simulink model "autoquet_simulink_expo_model"  (R2023b)
settings: Solver=FixedStepAuto  StartTime=0.0  StopTime=600  FixedStep=1e-4  RelTol=1e-3  EnableMultiTasking=on
libraries: svdutilitieslib x20, arduinolib x12, dspfdesign x2, arduinosensorlib x1
settings Model: ExtModeTrigDuration=2  Creator=doria  LastModifiedBy=doria
settings OptimizationCC: BlockReduction=off  EnhancedBackFolding=on  PassReuseOutputArgsAs=Individual arguments  ZeroExternalMemoryAtStartup=off  ZeroInternalMemoryAtStartup=off  MaxStackSize=64  OptimizeBlockOrder=speed  DifferentSizesBufferReuse=on  OptimizationCustomize=off  EfficientTunableParamExpr=on
settings DebuggingCC: MultiTaskCondExecSysMsg=warning  MultiTaskRateTransMsg=warning  ParameterTunabilityLossMsg=error
settings HardwareCC: ProdBitPerInt=16  ProdBitPerPointer=16  ProdBitPerSizeT=16  ProdBitPerPtrDiffT=16  ProdLargestAtomicFloat=None  ProdWordSize=8  ProdHWDeviceType=Atmel->AVR
settings ModelReferenceCC: UpdateModelReferenceTargets=Force
settings SFSimCC: MATLABDynamicMemAlloc=off
settings RTWCC: Description=Embedded Coder  SystemTargetFile=ert.tlc  HardwareBoard=Arduino Micro  TemplateMakefile=ert_default_tmf  Toolchain=Arduino AVR  BuildConfiguration=Faster Runs
settings CodeAppCC: ForceParamTrailComments=on  IgnoreCustomStorageClasses=off  OperatorAnnotations=on  SimulinkDataObjDesc=on  SFDataObjDesc=on  InsertBlockDesc=on
settings ERTTargetCC: SupportContinuousTime=on  SupportVariableSizeSignals=on  ExtModeTransport=3  ExtModeStaticAlloc=on  ExtModeAutomaticAllocSize=off  ExtModeStaticAllocSize=250  ExtModeMexFile=ext_xcp  ExtModeIntrfLevel=Level2 - Open

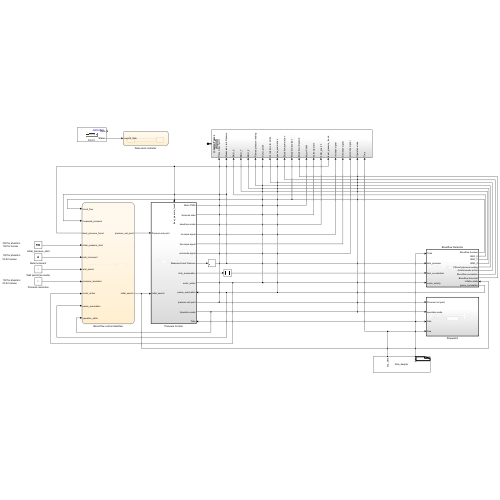
[thumbnail: Simulink's stored preview of the top-level diagram]
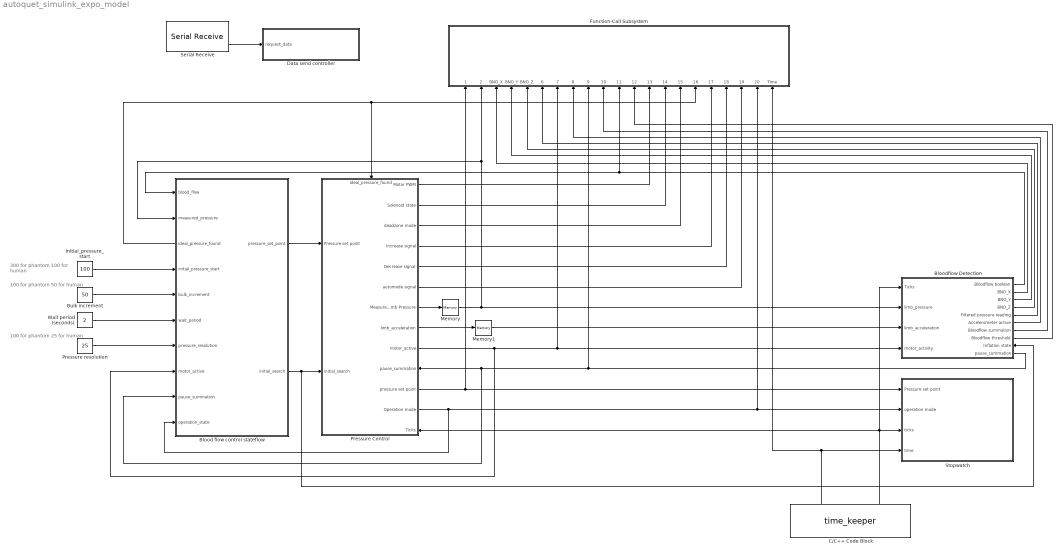
== system autoquet_simulink_expo_model ==
  note: 100 for phantom
      | 25 for human
  note: 100 for phantom
      | 50 for human
  note: 300 for phantom
      | 100 for human
  Blood flow control stateflow : Stateflow chart  TreatAsAtomicUnit=on
      settings: PortSchema="{\"entries\":[{\"content\":{\"sides\":[{\"content\":{\"connectorIds\":[\"In1\",\"In2\",\"Out3\",\"In4\",\"In5\",\"In6\",\"In7\",\"In3\",\"In9\",\"In8\"]},\"type\":\"ConnectorPlacement.EquallySpacedRectSide\",\"uuid\":\"812cdb75-6571-43e2-adf4-343057f083b7\"},{\"content\":{\"connectorIds\":[\"Out1\",\"Out2\"],\"side\":\"RIGHT\"},\"type\":\"ConnectorPlacement.EquallySpacedRectSide\",\"uuid\":\"a4b61973-6b2d-420b-b349-462770cb6915\"},{\"content\":{\"side\":\"TOP\"},\"type\":\"ConnectorPlacement.EquallySpacedRectSide\",\"uuid\":\"df2e293f-82b1-482e-98b7-6670b47b2c1c\"}]},\"type\":\"ConnectorPlacement.EquallySpacedConnector\",\"uuid\":\"fd5e7a3b-f236-4f3b-9c02-917a8b73c0b8\"}],\"packageUris\":[\"http://schema.mathworks.com/mf0/Connector/R2020b\"],\"version\":\"1.0\"}"
  Bloodflow Detection : Subsystem  TreatAsAtomicUnit=on
      settings: PortSchema="{\"entries\":[{\"content\":{\"sides\":[{\"content\":{\"connectorIds\":[\"In1\",\"In2\",\"In3\",\"In4\"]},\"type\":\"ConnectorPlacement.EquallySpacedRectSide\",\"uuid\":\"5e0e8b27-4c56-4ccb-b0a1-062650fc9649\"},{\"content\":{\"connectorIds\":[\"Out1\",\"Out2\",\"Out3\",\"Out4\",\"Out5\",\"Out6\",\"Out7\",\"Out8\",\"In5\",\"Out9\"],\"side\":\"RIGHT\"},\"type\":\"ConnectorPlacement.EquallySpacedRectSide\",\"uuid\":\"7358a381-cedb-4f62-990c-8a25243812b5\"},{\"content\":{\"side\":\"TOP\"},\"type\":\"ConnectorPlacement.EquallySpacedRectSide\",\"uuid\":\"a0c59af8-aeee-4320-9b7e-602a20d8920c\"}]},\"type\":\"ConnectorPlacement.EquallySpacedConnector\",\"uuid\":\"57543b81-d36e-431f-a997-66da3d45fb72\"}],\"packageUris\":[\"http://schema.mathworks.com/mf0/Connector/R2020b\"],\"version\":\"1.0\"}"
  Bulk increment : Constant  Value=50  OutDataTypeStr=single
  C/C++ Code Block : S-Function  FunctionName=time_keeper  SFunctionModules=time_keeper_wrapper.c  SFunctionDeploymentMode=off  EnableBusSupport=off  mask(S-Function Builder){}
      mask help: Simulink:masks:SFunctionBuilder_MD
      mask init:
      | val = [[.9  0.75 0.75 1 1 .9 .9 1]',[1 1 0.75 0.75 .9 .9 1 .9]'];try , sys = get_param(gcb,'SfunBuilderFcnName');if isempty(sys), sys = get_param(gcb,'FunctionName'); end,catch, sys = get_param(gcb,'FunctionName'); end
      settings: CopyFcn=set_param(gcbh,'LinkStatus','none')  OpenFcn=sfunctionwizard(gcbh)
      mask Display:
      | plot(val(:,1),val(:,2))
      | disp(sys)
      | port_label('output',1,'my_time')
      | port_label('output',2,'ticks')
  Data send controller : Stateflow chart  TreatAsAtomicUnit=on
  Function-Call Subsystem : Subsystem  TreatAsAtomicUnit=on
  Initial_pressure_start : Constant  Value=100  OutDataTypeStr=single
  Memory : Memory  InheritSampleTime=on  LinearizeAsDelay=on
  Memory1 : Memory  InheritSampleTime=on  LinearizeAsDelay=on
  Pressure Control : Subsystem  TreatAsAtomicUnit=on
      settings: PortSchema="{\"entries\":[{\"content\":{\"sides\":[{\"content\":{\"connectorIds\":[\"In1\",\"In2\"]},\"type\":\"ConnectorPlacement.EquallySpacedRectSide\",\"uuid\":\"ed00d6be-1556-4e99-a948-01e03a5de8aa\"},{\"content\":{\"connectorIds\":[\"Out1\",\"Out2\",\"Out3\",\"Out4\",\"Out5\",\"Out6\",\"Out7\",\"Out8\",\"Out9\",\"In4\",\"Out10\",\"Out11\",\"In5\"],\"side\":\"RIGHT\"},\"type\":\"ConnectorPlacement.EquallySpacedRectSide\",\"uuid\":\"cb154fea-e288-4b20-b221-160466b8fd95\"},{\"content\":{\"connectorIds\":[\"In3\"],\"side\":\"TOP\"},\"type\":\"ConnectorPlacement.EquallySpacedRectSide\",\"uuid\":\"7383458d-f718-4675-a86d-a540a43d0070\"},{\"content\":{\"side\":\"BOTTOM\"},\"type\":\"ConnectorPlacement.EquallySpacedRectSide\",\"uuid\":\"c6eee0b0-5b3b-4969-8554-67d16bbf2db7\"}]},\"type\":\"ConnectorPlacement.EquallySpacedConnector\",\"uuid\":\"fee8b448-539b-41ae-8871-4f9b2da6cd4e\"}],\"packageUris\":[\"http://schema.mathworks.com/mf0/Connector/R2020b\"],\"version\":\"1.0\"}"
  Pressure resolution : Constant  Value=25  OutDataTypeStr=single
  Serial Receive : arduinolib/Serial Receive  isARMArch=off  portNumber=0  DataType=uint8  Datalength=1  SampleTime=0.1  showOutStatus=on  blockPlatform=arduino
  Stopwatch : Subsystem  TreatAsAtomicUnit=on
  Wait period (seconds) : Constant  Value=2  OutDataTypeStr=single
  wires:
  Bloodflow Detection/3(BNO_Y) -> Function-Call Subsystem/4(BNO_Y)
  Bloodflow Detection/6(Accelerometer active) -> Function-Call Subsystem/8(Accelerometer active)
  Bloodflow Detection/5(Filtered pressure reading) -> Function-Call Subsystem/6(Filtered pressure reading)
  Bulk increment/1 -> Blood flow control stateflow/5(bulk_increment)
  Bloodflow Detection/8(Bloodflow threshold) -> Function-Call Subsystem/12(Bloodflow threshold)
  Pressure Control/8(limb_acceleration) -> Memory1/1
  Wait period (seconds)/1 -> Blood flow control stateflow/6(wait_period)
  Pressure Control/1(Motor PWM) -> Function-Call Subsystem/13(Motor PWM)
  Blood flow control stateflow/2(initial_search) -> Bloodflow Detection/5(Inflation state), Pressure Control/2(initial_search)
  Blood flow control stateflow/1(pressure_set_point) -> Pressure Control/1(Pressure set point)
  Initial_pressure_start/1 -> Blood flow control stateflow/4(initial_pressure_start)
  C/C++ Code Block/2 -> Bloodflow Detection/1(Ticks), Stopwatch/3(ticks), Pressure Control/5(Ticks)
  Pressure resolution/1 -> Blood flow control stateflow/7(pressure_resolution)
  Blood flow control stateflow/3(ideal_pressure_found) -> Function-Call Subsystem/16(ideal_pressure_found), Pressure Control/3(ideal_pressure_found)
  Bloodflow Detection/4(BNO_Z) -> Function-Call Subsystem/5(BNO_Z)
  Bloodflow Detection/2(BNO_X) -> Function-Call Subsystem/3(BNO_X)
  Pressure Control/6(automode signal) -> Function-Call Subsystem/19(automode signal)
  Pressure Control/3(deadzone mode) -> Function-Call Subsystem/15(initial_search)
  Pressure Control/2(Solenoid state) -> Function-Call Subsystem/14(Solenoid state)
  Bloodflow Detection/1(Bloodflow boolean) -> Function-Call Subsystem/11(Bloodflow boolean), Blood flow control stateflow/1(blood_flow)
  C/C++ Code Block/1 -> Function-Call Subsystem/21(Time), Stopwatch/4(time)
  Pressure Control/5(Decrease signal) -> Function-Call Subsystem/18(Decrease signal)
  Bloodflow Detection/7(Bloodflow summation) -> Function-Call Subsystem/10(Bloodflow summation)
  Pressure Control/4(Increase signal) -> Function-Call Subsystem/17(Increase signal)
  Pressure Control/10(pressure set point) -> Function-Call Subsystem/1(Pressure set point), Stopwatch/1(Pressure set point)
  Pressure Control/11(Operation mode) -> Blood flow control stateflow/8(operation_state), Function-Call Subsystem/20(Operation mode), Stopwatch/2(operation mode)
  Pressure Control/7(Measured Limb Pressure) -> Memory/1
  Pressure Control/9(motor_active) -> Blood flow control stateflow/3(motor_active), Function-Call Subsystem/7(motor_active), Bloodflow Detection/4(motor_activity)
  Bloodflow Detection/9(pause_summation) -> Function-Call Subsystem/9(pause_summation), Pressure Control/4(pause_summation), Blood flow control stateflow/9(pause_summation)
  Memory/1 -> Function-Call Subsystem/2(Measured Limb Pressure), Blood flow control stateflow/2(measured_pressure), Bloodflow Detection/2(limb_pressure)
  Memory1/1 -> Bloodflow Detection/3(limb_acceleration)
  Serial Receive/2 -> Data send controller/1(request_data)

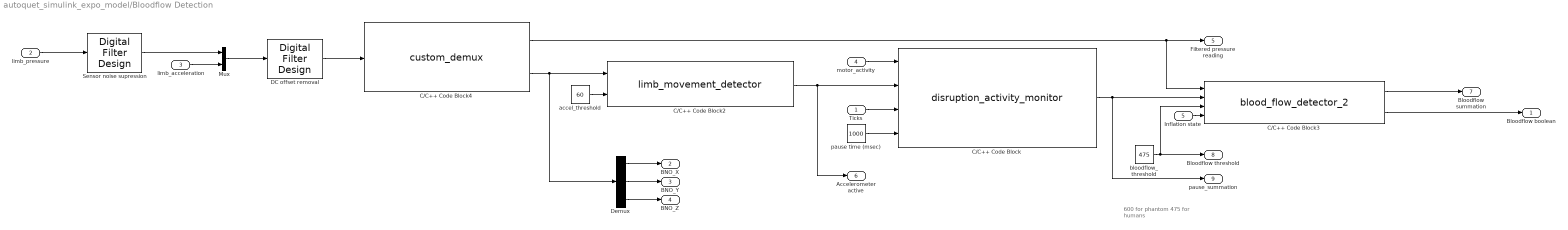
== system autoquet_simulink_expo_model/Bloodflow Detection ==
  note: 600 for phantom
      | 475 for humans
  Ticks : Inport
  limb_pressure : Inport  Port=2
  limb_acceleration : Inport  Port=3
  motor_activity : Inport  Port=4
  Inflation state : Inport  Port=5
  C/C++ Code Block : S-Function  FunctionName=disruption_activity_monitor  SFunctionModules=disruption_activity_monitor_wrapper.c  SFunctionDeploymentMode=off  EnableBusSupport=off  mask(S-Function Builder){}
      mask help: Simulink:masks:SFunctionBuilder_MD
      mask init: same as autoquet_simulink_expo_model/C/C++ Code Block
      settings: CopyFcn=set_param(gcbh,'LinkStatus','none')  OpenFcn=sfunctionwizard(gcbh)
      mask Display:
      | plot(val(:,1),val(:,2))
      | disp(sys)
      | port_label('input',1,'motor_active')
      | port_label('input',2,'movement_detected')
      | port_label('input',3,'time')
      | port_label('input',4,'pause_time')
      | port_label('output',1,'pause_summation')
  C/C++ Code Block2 : S-Function  FunctionName=limb_movement_detector  SFunctionModules=limb_movement_detector_wrapper.c  SFunctionDeploymentMode=off  EnableBusSupport=off  mask(S-Function Builder){}
      mask help: Simulink:masks:SFunctionBuilder_MD
      mask init: same as autoquet_simulink_expo_model/C/C++ Code Block
      settings: CopyFcn=set_param(gcbh,'LinkStatus','none')  OpenFcn=sfunctionwizard(gcbh)
      mask Display:
      | plot(val(:,1),val(:,2))
      | disp(sys)
      | port_label('input',1,'limb_acceleration')
      | port_label('input',2,'accel_threshold')
      | port_label('output',1,'movement_boolean')
  C/C++ Code Block3 : S-Function  FunctionName=blood_flow_detector_2  SFunctionModules=blood_flow_detector_2_wrapper.c  SFunctionDeploymentMode=off  EnableBusSupport=off  mask(S-Function Builder){}
      mask help: Simulink:masks:SFunctionBuilder_MD
      mask init: same as autoquet_simulink_expo_model/C/C++ Code Block
      settings: CopyFcn=set_param(gcbh,'LinkStatus','none')  OpenFcn=sfunctionwizard(gcbh)
      mask Display:
      | plot(val(:,1),val(:,2))
      | disp(sys)
      | port_label('input',1,'u0')
      | port_label('input',2,'disruption_active')
      | port_label('input',3,'bloodflow_threshold')
      | port_label('input',4,'inflation_state')
      | port_label('output',1,'y0')
      | port_label('output',2,'bloodflow_boolean')
  C/C++ Code Block4 : S-Function  FunctionName=custom_demux  SFunctionModules=custom_demux_wrapper.c  SFunctionDeploymentMode=off  EnableBusSupport=off  mask(S-Function Builder){}
      mask help: Simulink:masks:SFunctionBuilder_MD
      mask init: same as autoquet_simulink_expo_model/C/C++ Code Block
      settings: CopyFcn=set_param(gcbh,'LinkStatus','none')  OpenFcn=sfunctionwizard(gcbh)
      mask Display:
      | plot(val(:,1),val(:,2))
      | disp(sys)
      | port_label('input',1,'combined_vector')
      | port_label('output',1,'filtered_pressure')
      | port_label('output',2,'filtered_acceleration')
  DC offset removal : dspfdesign/Digital Filter Design  mwdsp_browser_bugfix_var=off
  Demux : Demux  Outputs=3
  Mux : Mux  Inputs=2
  Sensor noise supression : dspfdesign/Digital Filter Design  mwdsp_browser_bugfix_var=off
  accel_threshold : Constant  Value=60  OutDataTypeStr=uint16
  bloodflow_threshold : Constant  Value=475  OutDataTypeStr=uint16
  pause time (msec) : Constant  Value=1000  OutDataTypeStr=uint16
  Bloodflow boolean : Outport
  BNO_X : Outport  Port=2
  BNO_Y : Outport  Port=3
  BNO_Z : Outport  Port=4
  Filtered pressure reading : Outport  Port=5
  Accelerometer active : Outport  Port=6
  Bloodflow summation : Outport  Port=7
  Bloodflow threshold : Outport  Port=8
  pause_summation : Outport  Port=9
  wires:
  Mux/1 -> DC offset removal/1
  C/C++ Code Block3/2 -> Bloodflow boolean/1
  C/C++ Code Block3/1 -> Bloodflow summation/1
  accel_threshold/1 -> C/C++ Code Block2/2
  limb_pressure/1 -> Sensor noise supression/1
  Sensor noise supression/1 -> Mux/1
  DC offset removal/1 -> C/C++ Code Block4/1
  limb_acceleration/1 -> Mux/2
  C/C++ Code Block4/1 -> Filtered pressure reading/1, C/C++ Code Block3/1
  C/C++ Code Block4/2 -> C/C++ Code Block2/1, Demux/1
  Demux/1 -> BNO_X/1
  Demux/2 -> BNO_Y/1
  Demux/3 -> BNO_Z/1
  C/C++ Code Block2/1 -> Accelerometer active/1, C/C++ Code Block/2
  Ticks/1 -> C/C++ Code Block/3
  pause time (msec)/1 -> C/C++ Code Block/4
  motor_activity/1 -> C/C++ Code Block/1
  C/C++ Code Block/1 -> pause_summation/1, C/C++ Code Block3/2
  bloodflow_threshold/1 -> Bloodflow threshold/1, C/C++ Code Block3/3
  Inflation state/1 -> C/C++ Code Block3/4

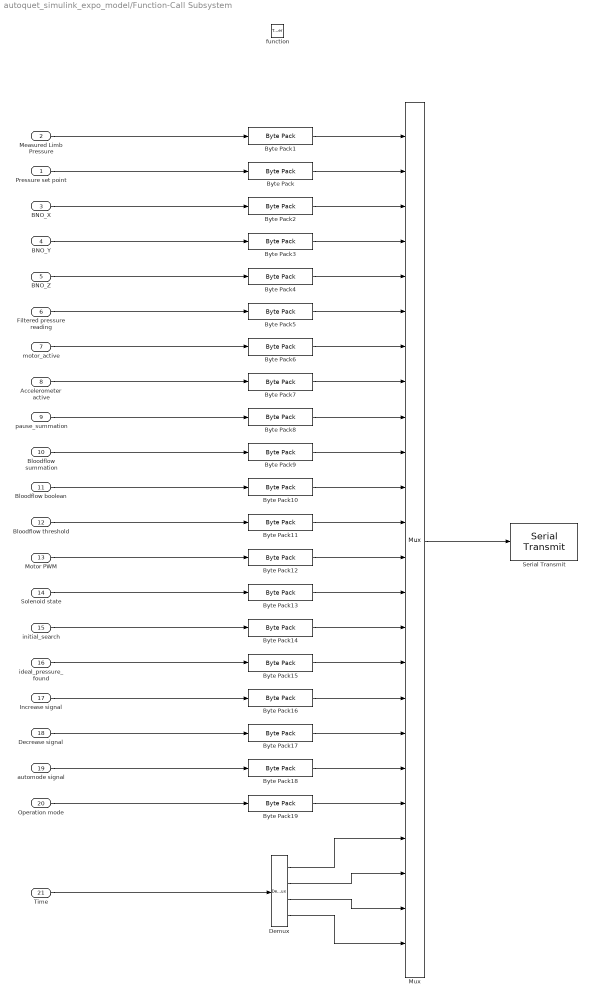
== system autoquet_simulink_expo_model/Function-Call Subsystem ==
  Pressure set point : Inport
  Measured Limb Pressure : Inport  Port=2
  BNO_X : Inport  Port=3
  BNO_Y : Inport  Port=4
  BNO_Z : Inport  Port=5
  Filtered pressure reading : Inport  Port=6
  motor_active : Inport  Port=7
  Accelerometer active : Inport  Port=8
  pause_summation : Inport  Port=9
  Bloodflow summation : Inport  Port=10
  Bloodflow boolean : Inport  Port=11
  Bloodflow threshold : Inport  Port=12
  Motor PWM : Inport  Port=13
  Solenoid state : Inport  Port=14
  initial_search : Inport  Port=15
  ideal_pressure_found : Inport  Port=16
  Increase signal : Inport  Port=17
  Decrease signal : Inport  Port=18
  automode signal : Inport  Port=19
  Operation mode : Inport  Port=20
  Time : Inport  Port=21
  function : TriggerPort  TriggerType=function-call  IsSimulinkFunction=on  FunctionName=send_params  VariantControl=(inherit)
  Byte Pack{,1..5,12} (7 alike) : svdutilitieslib/Byte Pack  maskPackedDataType=uint8  datatypes={'single'}  byteAlign=1  blockPlatform=arduinoert
  Byte Pack{6..8,10,13,15..18} (9 alike) : svdutilitieslib/Byte Pack  maskPackedDataType=uint8  datatypes={'boolean'}  byteAlign=1  blockPlatform=arduinoert
  Byte Pack11 : svdutilitieslib/Byte Pack  maskPackedDataType=uint8  datatypes={'uint16'}  byteAlign=1  blockPlatform=arduinoert
  Byte Pack14 : svdutilitieslib/Byte Pack  maskPackedDataType=uint8  datatypes={'uint8'}  byteAlign=1  blockPlatform=arduinoert
  Byte Pack19 : svdutilitieslib/Byte Pack  maskPackedDataType=uint8  datatypes={'uint8'}  byteAlign=1  blockPlatform=arduinoert
  Byte Pack9 : svdutilitieslib/Byte Pack  maskPackedDataType=uint8  datatypes={'uint16'}  byteAlign=1  blockPlatform=arduinoert
  Demux : Demux
  Mux : Mux  Inputs=24
  Serial Transmit : arduinolib/Serial Transmit  portNumber=0  sendmode=write  sendformat=Decimal  floatprecision=2  blockPlatform=arduino
  wires:
  Byte Pack19/1 -> Mux/20
  Solenoid state/1 -> Byte Pack13/1
  Bloodflow summation/1 -> Byte Pack9/1
  Operation mode/1 -> Byte Pack19/1
  Byte Pack18/1 -> Mux/19
  Increase signal/1 -> Byte Pack16/1
  Byte Pack/1 -> Mux/2
  Byte Pack13/1 -> Mux/14
  Demux/3 -> Mux/23
  Byte Pack17/1 -> Mux/18
  Time/1 -> Demux/1
  Demux/2 -> Mux/22
  Demux/1 -> Mux/21
  Byte Pack2/1 -> Mux/3
  BNO_Y/1 -> Byte Pack3/1
  Byte Pack11/1 -> Mux/12
  Measured Limb Pressure/1 -> Byte Pack1/1
  Accelerometer active/1 -> Byte Pack7/1
  Bloodflow threshold/1 -> Byte Pack11/1
  Byte Pack12/1 -> Mux/13
  Mux/1 -> Serial Transmit/1
  Decrease signal/1 -> Byte Pack17/1
  Pressure set point/1 -> Byte Pack/1
  Byte Pack15/1 -> Mux/16
  initial_search/1 -> Byte Pack14/1
  ideal_pressure_found/1 -> Byte Pack15/1
  Byte Pack9/1 -> Mux/10
  Byte Pack8/1 -> Mux/9
  Byte Pack1/1 -> Mux/1
  Byte Pack7/1 -> Mux/8
  pause_summation/1 -> Byte Pack8/1
  Byte Pack6/1 -> Mux/7
  motor_active/1 -> Byte Pack6/1
  automode signal/1 -> Byte Pack18/1
  Filtered pressure reading/1 -> Byte Pack5/1
  BNO_Z/1 -> Byte Pack4/1
  Bloodflow boolean/1 -> Byte Pack10/1
  BNO_X/1 -> Byte Pack2/1
  Byte Pack16/1 -> Mux/17
  Byte Pack10/1 -> Mux/11
  Byte Pack4/1 -> Mux/5
  Byte Pack14/1 -> Mux/15
  Motor PWM/1 -> Byte Pack12/1
  Byte Pack3/1 -> Mux/4
  Demux/4 -> Mux/24
  Byte Pack5/1 -> Mux/6

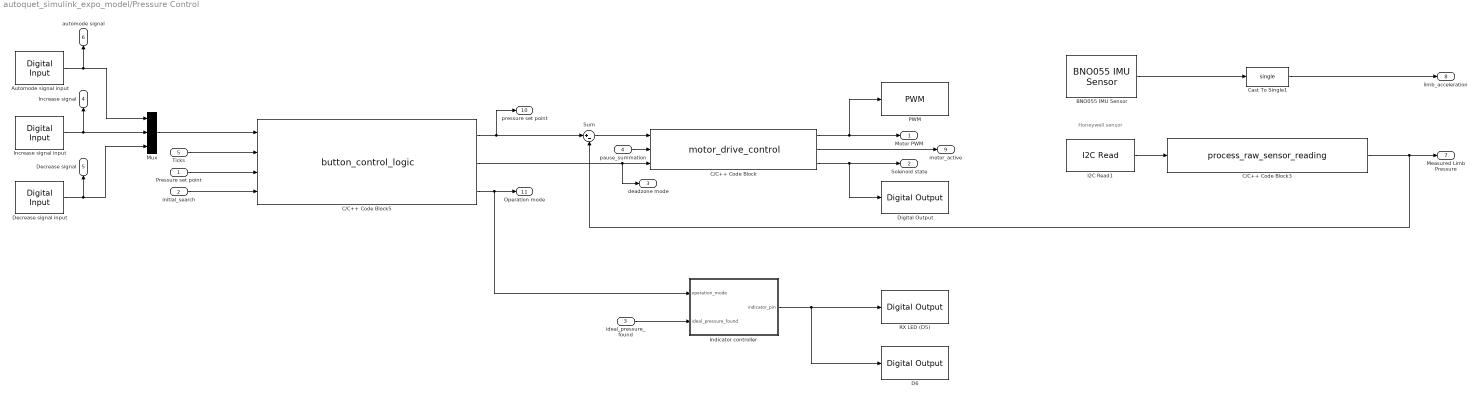
== system autoquet_simulink_expo_model/Pressure Control ==
  note: Honeywell sensor
  Pressure set point : Inport
  initial_search : Inport  Port=2
  ideal_pressure_found : Inport  Port=3
  pause_summation : Inport  Port=4
  Ticks : Inport  Port=5
  Automode signal input : arduinolib/Digital Input  pinNumber=0  mode=Default  Direction=input  SampleTime=-1  blockPlatform=arduino
  BNO055 IMU Sensor : arduinosensorlib/BNO055 IMU Sensor  SlaveAddress=0x29  OperationMode=Fusion  Accel=on  AngularRate=off  MagField=off  EulerAngles=off  Quat=off  LinearAccel=off  GravityVector=off  Status=off  Timestamp=off  AccelRange=4G  AccelBW=62.5 Hz  GyroRange=2000 dps  GyroBW=32 Hz  MagODR=10 Hz  spf=1  SampleTime=0.1  blockPlatform=ARDUINO  QueueSizeFactor=1
  C/C++ Code Block : S-Function  FunctionName=motor_drive_control  SFunctionModules=motor_drive_control_wrapper.c  SFunctionDeploymentMode=off  EnableBusSupport=off  mask(S-Function Builder){}
      mask help: Simulink:masks:SFunctionBuilder_MD
      mask init: same as autoquet_simulink_expo_model/C/C++ Code Block
      settings: CopyFcn=set_param(gcbh,'LinkStatus','none')  OpenFcn=sfunctionwizard(gcbh)
      mask Display:
      | plot(val(:,1),val(:,2))
      | disp(sys)
      | port_label('input',1,'limb_pressure_diff')
      | port_label('input',2,'pause_summation')
      | port_label('input',3,'initial_search')
      | port_label('output',1,'inflation_state')
      | port_label('output',2,'motor_active')
      | port_label('output',3,'solenoid_state')
  C/C++ Code Block3 : S-Function  FunctionName=process_raw_sensor_reading  SFunctionModules=process_raw_sensor_reading_wrapper.c  SFunctionDeploymentMode=off  EnableBusSupport=off  mask(S-Function Builder){}
      mask help: Simulink:masks:SFunctionBuilder_MD
      mask init: same as autoquet_simulink_expo_model/C/C++ Code Block
      settings: CopyFcn=set_param(gcbh,'LinkStatus','none')  OpenFcn=sfunctionwizard(gcbh)
      mask Display:
      | plot(val(:,1),val(:,2))
      | disp(sys)
      | port_label('input',1,'raw_sensor_input')
      | port_label('output',1,'limb_pressure_mmhg')
  C/C++ Code Block5 : S-Function  FunctionName=button_control_logic  SFunctionModules=button_control_logic_wrapper.c  SFunctionDeploymentMode=off  EnableBusSupport=off  mask(S-Function Builder){}
      mask help: Simulink:masks:SFunctionBuilder_MD
      mask init: same as autoquet_simulink_expo_model/C/C++ Code Block
      settings: CopyFcn=set_param(gcbh,'LinkStatus','none')  OpenFcn=sfunctionwizard(gcbh)
      mask Display:
      | plot(val(:,1),val(:,2))
      | disp(sys)
      | port_label('input',1,'button_signals')
      | port_label('input',2,'time')
      | port_label('input',3,'auto_pressure_setpoint')
      | port_label('input',4,'initial_search')
      | port_label('output',1,'pressure_set_point')
      | port_label('output',2,'roughness')
      | port_label('output',3,'operation_mode')
  Cast To Single1 : DataTypeConversion  OutDataTypeStr=single  SaturateOnIntegerOverflow=off  RndMeth=Floor
  D6 : arduinolib/Digital Output  pinNumber=11  Direction=output  blockPlatform=arduino
  Decrease signal input : arduinolib/Digital Input  pinNumber=6  mode=Default  Direction=input  SampleTime=-1  blockPlatform=arduino
  Digital Output : arduinolib/Digital Output  pinNumber=10  Direction=output  blockPlatform=arduino
  I2C Read1 : arduinolib/I2C Read  I2CModule=0  Mode=Master  SlaveAddress=0x28  SlaveByteOrder=BigEndian  Direction=Receiver  RegisterAddressMode=off  RegisterAddress=1  SlaveDataType=uint8  DataLength=2  NoAck=off  RepeatedStart=off  OutputStatus=off  blockPlatform=ARDUINO  SampleTime=0.1
  Increase signal input : arduinolib/Digital Input  pinNumber=4  mode=Default  Direction=input  SampleTime=-1  blockPlatform=arduino
  Indicator controller : Stateflow chart  TreatAsAtomicUnit=on
      settings: PortSchema="{\"entries\":[{\"content\":{\"sides\":[{\"content\":{\"connectorIds\":[\"In2\",\"In1\"]},\"type\":\"ConnectorPlacement.EquallySpacedRectSide\",\"uuid\":\"c5b6b3e1-eccf-47c2-ab3e-62c3b022a70b\"},{\"content\":{\"connectorIds\":[\"Out1\"],\"side\":\"RIGHT\"},\"type\":\"ConnectorPlacement.EquallySpacedRectSide\",\"uuid\":\"80991faa-c7f7-4917-af08-fc1f01769844\"},{\"content\":{\"side\":\"TOP\"},\"type\":\"ConnectorPlacement.EquallySpacedRectSide\",\"uuid\":\"8216009b-fd92-42a2-99c0-c5a03d94ecce\"}]},\"type\":\"ConnectorPlacement.EquallySpacedConnector\",\"uuid\":\"2e60610f-ceb9-47b9-b30e-e39dead51fee\"}],\"packageUris\":[\"http://schema.mathworks.com/mf0/Connector/R2020b\"],\"version\":\"1.0\"}"
  Mux : Mux  Inputs=3
  PWM : arduinolib/PWM  pinNumber=5  frequencyType=Default  desiredFrequency=490.2  achievableFrequency=490.2
  RX LED (D5) : arduinolib/Digital Output  pinNumber=17  Direction=output  blockPlatform=arduino
  Sum : Sum  Inputs=|+-
  Motor PWM : Outport
  Solenoid state : Outport  Port=2
  deadzone mode : Outport  Port=3
  Increase signal : Outport  Port=4
  Decrease signal : Outport  Port=5
  automode signal : Outport  Port=6
  Measured Limb Pressure : Outport  Port=7
  limb_acceleration : Outport  Port=8
  motor_active : Outport  Port=9
  pressure set point : Outport  Port=10
  Operation mode : Outport  Port=11
  wires:
  C/C++ Code Block3/1 -> Measured Limb Pressure/1, Sum/2
  I2C Read1/1 -> C/C++ Code Block3/1
  BNO055 IMU Sensor/1 -> Cast To Single1/1
  Cast To Single1/1 -> limb_acceleration/1
  Sum/1 -> C/C++ Code Block/1
  initial_search/1 -> C/C++ Code Block5/4
  Pressure set point/1 -> C/C++ Code Block5/3
  Ticks/1 -> C/C++ Code Block5/2
  Automode signal input/1 -> Mux/1, automode signal/1
  Increase signal input/1 -> Increase signal/1, Mux/2
  Decrease signal input/1 -> Mux/3, Decrease signal/1
  Mux/1 -> C/C++ Code Block5/1
  C/C++ Code Block5/3 -> Indicator controller/2(operation_mode), Operation mode/1
  C/C++ Code Block5/2 -> deadzone mode/1, C/C++ Code Block/3
  pause_summation/1 -> C/C++ Code Block/2
  C/C++ Code Block5/1 -> Sum/1, pressure set point/1
  C/C++ Code Block/1 -> PWM/1, Motor PWM/1
  C/C++ Code Block/3 -> Solenoid state/1, Digital Output/1
  C/C++ Code Block/2 -> motor_active/1
  ideal_pressure_found/1 -> Indicator controller/1(ideal_pressure_found)
  Indicator controller/1(indicator_pin) -> D6/1, RX LED (D5)/1

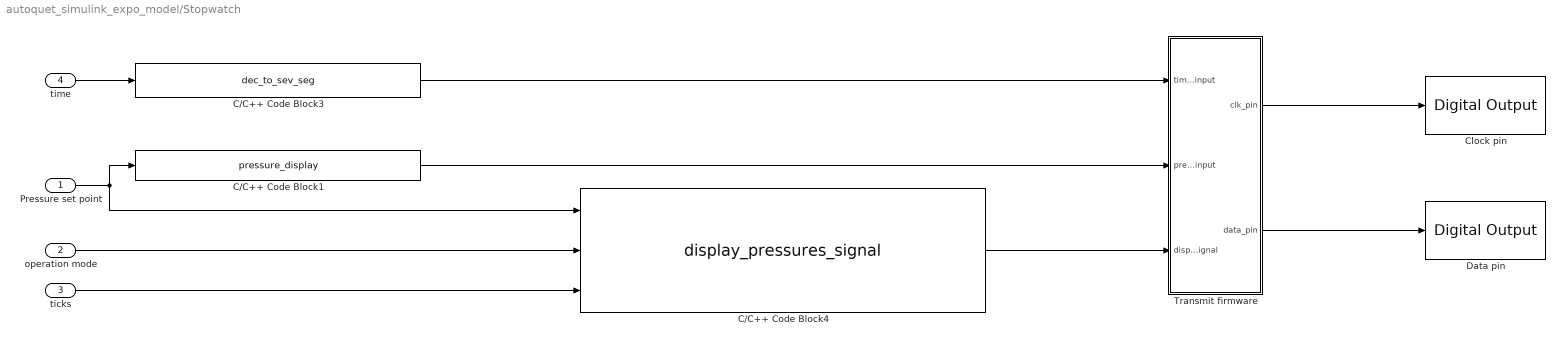
== system autoquet_simulink_expo_model/Stopwatch ==
  Pressure set point : Inport
  operation mode : Inport  Port=2
  ticks : Inport  Port=3
  time : Inport  Port=4
  C/C++ Code Block1 : S-Function  FunctionName=pressure_display  SFunctionModules=pressure_display_wrapper.c  SFunctionDeploymentMode=off  EnableBusSupport=off  mask(S-Function Builder){}
      mask help: Simulink:masks:SFunctionBuilder_MD
      mask init: same as autoquet_simulink_expo_model/C/C++ Code Block
      settings: CopyFcn=set_param(gcbh,'LinkStatus','none')  OpenFcn=sfunctionwizard(gcbh)
      mask Display:
      | plot(val(:,1),val(:,2))
      | disp(sys)
      | port_label('input',1,'set_point_pressure')
      | port_label('output',1,'digit_array')
  C/C++ Code Block3 : S-Function  FunctionName=dec_to_sev_seg  SFunctionModules=dec_to_sev_seg_wrapper.c  SFunctionDeploymentMode=off  EnableBusSupport=off  mask(S-Function Builder){}
      mask help: Simulink:masks:SFunctionBuilder_MD
      mask init: same as autoquet_simulink_expo_model/C/C++ Code Block
      settings: CopyFcn=set_param(gcbh,'LinkStatus','none')  OpenFcn=sfunctionwizard(gcbh)
      mask Display:
      | plot(val(:,1),val(:,2))
      | disp(sys)
      | port_label('input',1,'time_input')
      | port_label('output',1,'binary_time')
  C/C++ Code Block4 : S-Function  FunctionName=display_pressures_signal  SFunctionModules=display_pressures_signal_wrapper.c  SFunctionDeploymentMode=off  EnableBusSupport=off  mask(S-Function Builder){}
      mask help: Simulink:masks:SFunctionBuilder_MD
      mask init: same as autoquet_simulink_expo_model/C/C++ Code Block
      settings: CopyFcn=set_param(gcbh,'LinkStatus','none')  OpenFcn=sfunctionwizard(gcbh)
      mask Display:
      | plot(val(:,1),val(:,2))
      | disp(sys)
      | port_label('input',1,'pressure_set_point')
      | port_label('input',2,'operation_state')
      | port_label('input',3,'time')
      | port_label('output',1,'display_pressure_signal')
  Clock pin : arduinolib/Digital Output  pinNumber=8  Direction=output  blockPlatform=arduino
  Data pin : arduinolib/Digital Output  pinNumber=9  Direction=output  blockPlatform=arduino
  Transmit firmware : Stateflow chart  TreatAsAtomicUnit=on
      settings: PortSchema="{\"entries\":[{\"content\":{\"sides\":[{\"content\":{\"connectorIds\":[\"In1\",\"In3\",\"In2\"]},\"type\":\"ConnectorPlacement.EquallySpacedRectSide\",\"uuid\":\"1efc1697-0579-47d3-9fc4-5de77e3f0626\"},{\"content\":{\"connectorIds\":[\"Out1\",\"Out2\"],\"side\":\"RIGHT\"},\"type\":\"ConnectorPlacement.EquallySpacedRectSide\",\"uuid\":\"ff69e6e4-600f-4452-8192-a6d24cc22f95\"},{\"content\":{\"side\":\"TOP\"},\"type\":\"ConnectorPlacement.EquallySpacedRectSide\",\"uuid\":\"05ed7778-23b9-4edb-a8ad-4854108c3cad\"}]},\"type\":\"ConnectorPlacement.EquallySpacedConnector\",\"uuid\":\"b0f7e484-46c4-4185-b04a-c753f7ab6971\"}],\"packageUris\":[\"http://schema.mathworks.com/mf0/Connector/R2020b\"],\"version\":\"1.0\"}"
  wires:
  Transmit firmware/1(clk_pin) -> Clock pin/1
  Transmit firmware/2(data_pin) -> Data pin/1
  time/1 -> C/C++ Code Block3/1
  Pressure set point/1 -> C/C++ Code Block4/1, C/C++ Code Block1/1
  C/C++ Code Block1/1 -> Transmit firmware/3(pressure_input)
  operation mode/1 -> C/C++ Code Block4/2
  C/C++ Code Block4/1 -> Transmit firmware/2(display_signal)
  C/C++ Code Block3/1 -> Transmit firmware/1(time_input)
  ticks/1 -> C/C++ Code Block4/3

== stateflow chart autoquet_simulink_expo_model/Stopwatch/Transmit firmware ==
  state sending_firmware
    state send_data
      exit:
      clk_pin = true
      word_iterator = 1
      state data_high
        entry:
        data_pin = true
      state ack_bit
        entry:
        clk_pin = false
        exit:
        data_pin = false
      state latch_data
        entry:
        clk_pin = true
        buffer = bitshift(buffer, -1)
        bit_iterator = bit_iterator + 1
      state buffer_reset
        entry:
        buffer = to_screen(word_iterator-1)
        exit:
        bit_iterator = 1
      state reset_clk
        entry:
        clk_pin = false
      state post_ack_reset
        entry:
        word_iterator = word_iterator + 1
      state idler1
        exit:
        clk_pin = true
      state idler
        exit:
        clk_pin = false
      state data_low
        entry:
        data_pin = false
      reset_clk -> data_high [order 2] : [bitand(buffer, 1) == 1]
      data_high -> latch_data
      (default) -> reset_clk
      post_ack_reset -> buffer_reset : [word_iterator <= len]
      latch_data -> ack_bit [order 2] : [bit_iterator > 8]
      latch_data -> reset_clk [order 1] : [bit_iterator <= 8]
      buffer_reset -> reset_clk
      reset_clk -> data_low [order 1] : [bitand(buffer, 1) == 0]
      idler -> post_ack_reset
      data_low -> latch_data
      ack_bit -> idler1
      idler1 -> idler
    state Start_signal
      entry:
      data_pin = false
      buffer = command
      bit_iterator = 1
      word_iterator = 1
    state Stop
      entry:
      transmit = false
      exit:
      data_pin = true
    state init
      entry:
      command_state = 0
      transmit = false
      data_pin = true
      clk_pin = true
      full_data_sent = false
    state command_flow
      state find_command
      state transmit_data
        entry:
        command = 192
        len = 5
        command_state = command_state + 1
        transmit = true
      state data_directive
        entry:
        command = 64
        len = 1
        command_state = command_state + 1
        transmit = true
      state display_control
        entry:
        command = 136 %(Dimmest)
        %command = 143 %(Brightest)
        len = 1
        command_state = 0
        transmit = true
      (default) -> find_command
      find_command -> data_directive [order 1] : [command_state == 0]
      find_command -> transmit_data [order 2] : [command_state == 1]
      find_command -> display_control [order 3] : [command_state == 2]
    Start_signal -> send_data
    send_data -> Stop : [word_iterator >len]
    Stop -> command_flow [order 1] : [command ~= 136]
    Stop -> command_flow [order 2] : [command == 136]{full_data_sent = true}
    command_flow -> Start_signal : [transmit == true]
    (default) -> init
    init -> command_flow
  state set_time_to_display
    entry:
    to_screen = time_input
  state display_multiplexer
    flash_ratio = 7
  state set_pressure_to_display
    entry:
    to_screen = pressure_input
  state flashing_logic
    entry:
    pressure_flash = pressure_flash + 1
  state set_blank_to_display
    entry:
    to_screen = [0;0;0;0]
    pressure_flash = 0
  (default) -> display_multiplexer
  display_multiplexer -> set_time_to_display [order 2] : [display_signal == 0] % Display time
  set_time_to_display -> sending_firmware
  set_pressure_to_display -> sending_firmware
  flashing_logic -> set_pressure_to_display [order 1] : [rem(pressure_flash, flash_ratio) ~= 0]
  sending_firmware -> display_multiplexer : [full_data_sent == true]
  display_multiplexer -> flashing_logic [order 1] : [display_signal == 1] % Display pressure
  set_blank_to_display -> sending_firmware
  flashing_logic -> set_blank_to_display [order 2] : [rem(pressure_flash, flash_ratio) == 0]
  data: clk_pin output; data_pin output boolean; bit_iterator local uint8; buffer local uint8; len local uint8; word_iterator local uint8; time_input input uint8 size=[4,1]; command_state local uint8; command local uint8; to_screen local uint8 size=[4,1]; display_signal input uint8; pressure_input input uint8 size=[4,1]; full_data_sent local boolean; pressure_flash local uint8; transmit local boolean =false; flash_ratio local uint8

== stateflow chart autoquet_simulink_expo_model/Data send controller ==
  state wait
  state request_data
    entry:
    send_params();
  (default) -> wait
  wait -> request_data : [request_data == 1]
  request_data -> wait
  data: request_data input

== stateflow chart autoquet_simulink_expo_model/Blood flow control stateflow ==
  settings: updateMethod=DISCRETE  sampleTime=0.05
  state Manual_mode
    entry:
    initial_search = 3
  state Auto_mode
    state Binary_search_ideal_pressure
      % Find ideal pressure to stop bleeding between pressure extremes measured in previous stage
      entry:
      %binary_search_upper = 290 %pressure_upper_bound
      %binary_search_lower = 100 %pressure_lower_bound
      binary_search_upper = pressure_upper_bound
      binary_search_lower = pressure_lower_bound
      state Too_tight
        entry:
        binary_search_upper = pressure_set_point
      state Adjust_pressure_set_point
        entry:
        pressure_set_point = (binary_search_upper + binary_search_lower)/2
        pressure_difference = binary_search_upper - binary_search_lower
      state Ideal_pressure_found
        entry:
        pressure_set_point = binary_search_upper
        ideal_pressure_found = true
      state Idle
      state Too_loose
        entry:
        binary_search_lower = pressure_set_point
      Too_tight -> Adjust_pressure_set_point
      (junction 112) -> Too_tight [order 3] : [pressure_difference >= pressure_resolution ...
          |  && blood_flow == 0]
      (default) -> Adjust_pressure_set_point
      (junction 112) -> Ideal_pressure_found [order 1] : [pressure_difference < pressure_resolution]
      Auto_mode.Binary_search_ideal_pressure.Idle -> (junction 112) : [duration(motor_active == 0) > wait_period]
      Adjust_pressure_set_point -> Auto_mode.Binary_search_ideal_pressure.Idle : [(measured_pressure >= pressure_set_point - pressure_resolution/2) ...
          | && (measured_pressure  <= pressure_set_point + pressure_resolution/2) && pause_summation == 0]
      (junction 112) -> Too_loose [order 2] : [pressure_difference >= pressure_resolution ...
          |  && blood_flow > 0]
      Too_loose -> Adjust_pressure_set_point
    state Find_initial_bounds
      entry:
      pressure_set_point = initial_pressure_start
      upper_bound_found = false
      initial_search = 0
      ideal_pressure_found = false
      exit:
      initial_search = 2
      state Inflate
        %Inflate quickly to stop blood flow
        exit:
        pressure_upper_bound = pressure_set_point
        initial_search = 1
        state Increase_pressure_set_point
          entry:
          pressure_set_point = pressure_set_point + bulk_increment %bulk_increment
        state Idle
        state wait
        (default) -> wait
        Auto_mode.Find_initial_bounds.Inflate.Idle -> Increase_pressure_set_point : [duration(pause_summation == 0, sec) > 1.6*wait_period]
        wait -> Auto_mode.Find_initial_bounds.Inflate.Idle : [measured_pressure >= pressure_set_point]
        Increase_pressure_set_point -> wait
      state Deflate
        % Deflate until blood flow returns
        exit:
        pressure_lower_bound = pressure_set_point
        state Idle
        state Decrease_pressure_set_point
          entry:
          pressure_set_point = pressure_set_point - bulk_increment %bulk_decrement
        state Wait
        (default) -> Decrease_pressure_set_point
        Auto_mode.Find_initial_bounds.Deflate.Wait -> Auto_mode.Find_initial_bounds.Deflate.Idle : [measured_pressure<=pressure_set_point]
        Auto_mode.Find_initial_bounds.Deflate.Idle -> Decrease_pressure_set_point : [duration(pause_summation == 0) > wait_period]
        Decrease_pressure_set_point -> Auto_mode.Find_initial_bounds.Deflate.Wait
      (default) -> Inflate
      Inflate -> Deflate : [blood_flow == 0 && duration(pause_summation == 0, sec) > 1.5*wait_period]{upper_bound_found = true}
    state Steady_state
      entry:
      pressure_set_point = pressure_set_point + 50
      state Wait
      state slight_deflation
        entry:
        pressure_set_point = pressure_set_point - 100
      state re_inflate
        entry:
        pressure_set_point = pressure_set_point + 100
      (default) -> Auto_mode.Steady_state.Wait
      Auto_mode.Steady_state.Wait -> slight_deflation : after(300, sec)
      slight_deflation -> re_inflate : after(30, sec)
      re_inflate -> Auto_mode.Steady_state.Wait
    (default) -> Find_initial_bounds
    Binary_search_ideal_pressure -> Steady_state : [ideal_pressure_found==true]
    Find_initial_bounds -> Binary_search_ideal_pressure : [blood_flow > 0 && upper_bound_found == true]
  (default) -> Manual_mode
  Manual_mode -> Auto_mode : [operation_state == 1]
  Auto_mode -> Manual_mode : [operation_state == 0]
  data: pressure_set_point output single; blood_flow input; measured_pressure input single; binary_search_lower local single; binary_search_upper local single; pressure_difference local single; pressure_lower_bound local single; pressure_upper_bound local single; upper_bound_found local boolean; motor_active input boolean; initial_pressure_start input; bulk_increment input; wait_period input; pressure_resolution input; initial_search output uint8; ideal_pressure_found output boolean; operation_state input uint8; pause_summation input boolean

== stateflow chart autoquet_simulink_expo_model/Pressure Control/Indicator controller ==
  state Blink_indicator
    state led_on
      entry:
      indicator_pin = true
    state led_off
      entry:
      indicator_pin = false
    (default) -> led_off
    led_off -> led_on : after(200, msec)
    led_on -> led_off : after(200, msec)
  state Indicator_off
    entry:
    indicator_pin = false;
  state Solid_indicator
    entry:
    indicator_pin = true;
  (default) -> Indicator_off
  Blink_indicator -> Solid_indicator [order 1] : [duration(ideal_pressure_found == 1, msec) > 200]
  Indicator_off -> Blink_indicator : [operation_mode == 1]
  Solid_indicator -> (junction 10) : [operation_mode == 0]
  (junction 10) -> Indicator_off
  Blink_indicator -> (junction 10) [order 2] : [operation_mode == 0]
  data: ideal_pressure_found input boolean; operation_mode input uint8; indicator_pin output boolean
